simulink model "W02_Base_Map_PB_cs"  (R2019a)
settings: Solver=FixedStepDiscrete  StartTime=0.0  StopTime=inf  FixedStep=1/300  RelTol=1e-3
PreLoadFcn:
  | mbxruntime.callbacks.PreLoadFcn(bdroot);
  | check_NUTS_defined
  | model_closed = 0;
  | assignin('base',['model_closed_' bdroot],false);
PostLoadFcn:
  | mbxruntime.callbacks.PostLoadFcn(bdroot);
InitFcn:
  | mbxruntime.callbacks.InitFcn(bdroot);
StartFcn:
  | mbxruntime.callbacks.StartFcn(bdroot);
StopFcn:
  | mbxruntime.callbacks.StopFcn(bdroot);;
  | 
model workspace: external: MAT-File .\W02_Base_Map_PB_cs_hws.mat (data not in the file)
undefined symbols (not defined in the file or in its folder): DiscIntNeverNeededParam, Header, InitImageOutputDir, mbxruntime, Orientation, Pose, Poses, Poses_SL_Info, Position, tabledata
libraries: PBCSimulinkLibrary x57, simulink_extras x9, PreScanSimulinkLibrary x6, robotlib x6, PreScanUsefulBlocks x4, sharedtransform x3, aerolibutil x2, visionconversions x1, visionsinks x1
(part 4 of 7)

== system W02_Base_Map_PB_cs/TrafficLightRoadSideNL_7 ==
  note: Light SPD Resources
      |
      |  0: CIE_A_standard_incandescent_illuminant.txt
      |  1: CIE_A_standard_incandescent_illuminant.txt_x_R255_G191_B000.txt
      |  2: CIE_A_standard_incandescent_illuminant.txt_x_R583_G047_B000.txt
      |  3: CIE_F12_standard_fluorescent_illuminant.txt
      |  4: Illuminant_D65.txt
      |  5: Light_SPD_H1_12_8V_Filament.txt
      |  6: Light_SPD_H1_13_2V_Filament.txt
      |  7: Light_SPD_H11_12V_Filament.txt
      |  8: Light_SPD_H7_12_8V_Filament.txt
      |  9: Light_SPD_H7_13_2V_Filament.txt
      | 10: Light_SPD_H8_13_2V_Filament.txt
      | 11: Light_SPD_Halogen.txt
      | 12: Light_SPD_High_Power_LED.txt
      | 13: Light_SPD_HPS_High_Pressure_Sodium.txt
      | 14: Light_SPD_incandescent_traffic_signal_amber.txt
      | 15: Light_SPD_incandescent_traffic_signal_green.txt
      | 16: Light_SPD_incandescent_traffic_signal_red.txt
      | 17: Light_SPD_LED_D1S_HID.txt
      | 18: Light_SPD_LED_traffic_signal_amber.txt
      | 19: Light_SPD_LED_traffic_signal_green.txt
      | 20: Light_SPD_LED_traffic_signal_red.txt
      | 21: Light_SPD_LPS_Low_Pressure_Sodium.txt
      | 22: Light_SPD_Mercury.txt
      | 23: Light_SPD_Reddish_Neon_Sign.txt
      | 24: Noma_Twister_Blue_13W_120V.txt
      | 25: Philips_Blue_Golite_P1_Apollo_1750Lux.txt
      | 26: SPD_flat_1.0.txt
  note: Light SPD Resources
  Ground_1 : Ground
  Ground_2 : Ground
  Ground_3 : Ground
  TrafficLightRoadSideNL_7_Casing.LightGreen_Control_Mux : Subsystem  Tag=mux/plugin/LightSignals
  TrafficLightRoadSideNL_7_Casing.LightGreen_Power : Constant  Tag=TrafficLightRoadSideNL_7_Casing.LightGreen_Power  Value=0
  TrafficLightRoadSideNL_7_Casing.LightGreen_SPDIndex : Constant  Tag=TrafficLightRoadSideNL_7_Casing.LightGreen_SPDIndex  Value=15
  TrafficLightRoadSideNL_7_Casing.LightOrange_Control_Mux : Subsystem  Tag=mux/plugin/LightSignals
  TrafficLightRoadSideNL_7_Casing.LightOrange_Power : Constant  Tag=TrafficLightRoadSideNL_7_Casing.LightOrange_Power  Value=0
  TrafficLightRoadSideNL_7_Casing.LightOrange_SPDIndex : Constant  Tag=TrafficLightRoadSideNL_7_Casing.LightOrange_SPDIndex  Value=14
  TrafficLightRoadSideNL_7_Casing.LightRed_Control_Mux : Subsystem  Tag=mux/plugin/LightSignals
  TrafficLightRoadSideNL_7_Casing.LightRed_Power : Constant  Tag=TrafficLightRoadSideNL_7_Casing.LightRed_Power  Value=0
  TrafficLightRoadSideNL_7_Casing.LightRed_SPDIndex : Constant  Tag=TrafficLightRoadSideNL_7_Casing.LightRed_SPDIndex  Value=16
  VISUCasingLights_Mux : Subsystem  Tag=mux/VisuCasingLights  mask(PreScan User Interface: VisuTrafficLight){}
      mask help:
      | The VisuTrafficLight block provides a way to animate traffic lights: switch on and off individual lights.
      |
      | For more information, please click Help.
      mask Help: eval('openHelp(731)')
  VISUCasingLights_TrafficLightRoadSideNL_7 : Outport  Tag=outport/VisuCasingLights  SampleTime=1/300
  TrafficLightRoadSideNL_7_Casing.LightRed_Control : Outport  Tag=outport/plugin/sfun_PBCLight  Port=2  OutDataTypeStr=Bus: PRESCAN_PBCLIGHT_DATA  PortDimensions=1  SampleTime=0.05
  TrafficLightRoadSideNL_7_Casing.LightOrange_Control : Outport  Tag=outport/plugin/sfun_PBCLight  Port=3  OutDataTypeStr=Bus: PRESCAN_PBCLIGHT_DATA  PortDimensions=1  SampleTime=0.05
  TrafficLightRoadSideNL_7_Casing.LightGreen_Control : Outport  Tag=outport/plugin/sfun_PBCLight  Port=4  OutDataTypeStr=Bus: PRESCAN_PBCLIGHT_DATA  PortDimensions=1  SampleTime=0.05
  wires:
  VISUCasingLights_Mux/1(VISUCasingLights_TrafficLightRoadSideNL_7) -> VISUCasingLights_TrafficLightRoadSideNL_7/1
  TrafficLightRoadSideNL_7_Casing.LightRed_Control_Mux/1(Bus) -> TrafficLightRoadSideNL_7_Casing.LightRed_Control/1
  TrafficLightRoadSideNL_7_Casing.LightRed_SPDIndex/1 -> TrafficLightRoadSideNL_7_Casing.LightRed_Control_Mux/1(SPDIndex [-])
  TrafficLightRoadSideNL_7_Casing.LightRed_Power/1 -> TrafficLightRoadSideNL_7_Casing.LightRed_Control_Mux/2(Power [W])
  TrafficLightRoadSideNL_7_Casing.LightOrange_Control_Mux/1(Bus) -> TrafficLightRoadSideNL_7_Casing.LightOrange_Control/1
  TrafficLightRoadSideNL_7_Casing.LightOrange_SPDIndex/1 -> TrafficLightRoadSideNL_7_Casing.LightOrange_Control_Mux/1(SPDIndex [-])
  TrafficLightRoadSideNL_7_Casing.LightOrange_Power/1 -> TrafficLightRoadSideNL_7_Casing.LightOrange_Control_Mux/2(Power [W])
  TrafficLightRoadSideNL_7_Casing.LightGreen_Control_Mux/1(Bus) -> TrafficLightRoadSideNL_7_Casing.LightGreen_Control/1
  TrafficLightRoadSideNL_7_Casing.LightGreen_SPDIndex/1 -> TrafficLightRoadSideNL_7_Casing.LightGreen_Control_Mux/1(SPDIndex [-])
  TrafficLightRoadSideNL_7_Casing.LightGreen_Power/1 -> TrafficLightRoadSideNL_7_Casing.LightGreen_Control_Mux/2(Power [W])
  Ground_1/1 -> VISUCasingLights_Mux/1(Green [-])
  Ground_2/1 -> VISUCasingLights_Mux/2(Orange [-])
  Ground_3/1 -> VISUCasingLights_Mux/3(Red [-])

== system W02_Base_Map_PB_cs/TrafficLightRoadSideNL_7_Casing.LightGreen_Control ==
  TrafficLightRoadSideNL_7_Casing.LightGreen_Control : Inport  Tag=inport/plugin/sfun_PBCLight  OutDataTypeStr=Bus: PRESCAN_PBCLIGHT_DATA  PortDimensions=1  SampleTime=0.05  BusOutputAsStruct=on
  Actuator : S-Function  LoadFcn=addpath 'C:/Program Files/Simcenter Prescan/Prescan_2019.2/Plugins/PBCameraPlugin/matlab';addpath 'C:/Program Files/Simcenter Prescan/Prescan_2019.2/Plugins/PBCameraPlugin/bin';load('PreScanPBCLightData.mat');  FunctionName=sfun_PBCLight  Parameters=lightID, timestepMask  SFunctionDeploymentMode=off  EnableBusSupport=off  mask(Physics Based Camera plugin block){lightID=17, timestepMask=0.05}
      mask prompts: lightID "Light ID:"; timestepMask "MATLAB timestep:"
      mask help: Light Control I/O
      mask Help: eval('openHelp(6500)')
      mask Display: image(imread('ico_PBCControl.png'))
  wires:
  TrafficLightRoadSideNL_7_Casing.LightGreen_Control/1 -> Actuator/1

== system W02_Base_Map_PB_cs/TrafficLightRoadSideNL_7_Casing.LightOrange_Control ==
  TrafficLightRoadSideNL_7_Casing.LightOrange_Control : Inport  Tag=inport/plugin/sfun_PBCLight  OutDataTypeStr=Bus: PRESCAN_PBCLIGHT_DATA  PortDimensions=1  SampleTime=0.05  BusOutputAsStruct=on
  Actuator : S-Function  LoadFcn=addpath 'C:/Program Files/Simcenter Prescan/Prescan_2019.2/Plugins/PBCameraPlugin/matlab';addpath 'C:/Program Files/Simcenter Prescan/Prescan_2019.2/Plugins/PBCameraPlugin/bin';load('PreScanPBCLightData.mat');  FunctionName=sfun_PBCLight  Parameters=lightID, timestepMask  SFunctionDeploymentMode=off  EnableBusSupport=off  mask(Physics Based Camera plugin block){lightID=16, timestepMask=0.05}
      mask prompts: lightID "Light ID:"; timestepMask "MATLAB timestep:"
      mask help: Light Control I/O
      mask Help: eval('openHelp(6500)')
      mask Display: image(imread('ico_PBCControl.png'))
  wires:
  TrafficLightRoadSideNL_7_Casing.LightOrange_Control/1 -> Actuator/1

== system W02_Base_Map_PB_cs/TrafficLightRoadSideNL_7_Casing.LightRed_Control ==
  TrafficLightRoadSideNL_7_Casing.LightRed_Control : Inport  Tag=inport/plugin/sfun_PBCLight  OutDataTypeStr=Bus: PRESCAN_PBCLIGHT_DATA  PortDimensions=1  SampleTime=0.05  BusOutputAsStruct=on
  Actuator : S-Function  LoadFcn=addpath 'C:/Program Files/Simcenter Prescan/Prescan_2019.2/Plugins/PBCameraPlugin/matlab';addpath 'C:/Program Files/Simcenter Prescan/Prescan_2019.2/Plugins/PBCameraPlugin/bin';load('PreScanPBCLightData.mat');  FunctionName=sfun_PBCLight  Parameters=lightID, timestepMask  SFunctionDeploymentMode=off  EnableBusSupport=off  mask(Physics Based Camera plugin block){lightID=15, timestepMask=0.05}
      mask prompts: lightID "Light ID:"; timestepMask "MATLAB timestep:"
      mask help: Light Control I/O
      mask Help: eval('openHelp(6500)')
      mask Display: image(imread('ico_PBCControl.png'))
  wires:
  TrafficLightRoadSideNL_7_Casing.LightRed_Control/1 -> Actuator/1

== system W02_Base_Map_PB_cs/TrafficLightRoadSideNL_8 ==
  note: Light SPD Resources
      |
      |  0: CIE_A_standard_incandescent_illuminant.txt
      |  1: CIE_A_standard_incandescent_illuminant.txt_x_R255_G191_B000.txt
      |  2: CIE_A_standard_incandescent_illuminant.txt_x_R583_G047_B000.txt
      |  3: CIE_F12_standard_fluorescent_illuminant.txt
      |  4: Illuminant_D65.txt
      |  5: Light_SPD_H1_12_8V_Filament.txt
      |  6: Light_SPD_H1_13_2V_Filament.txt
      |  7: Light_SPD_H11_12V_Filament.txt
      |  8: Light_SPD_H7_12_8V_Filament.txt
      |  9: Light_SPD_H7_13_2V_Filament.txt
      | 10: Light_SPD_H8_13_2V_Filament.txt
      | 11: Light_SPD_Halogen.txt
      | 12: Light_SPD_High_Power_LED.txt
      | 13: Light_SPD_HPS_High_Pressure_Sodium.txt
      | 14: Light_SPD_incandescent_traffic_signal_amber.txt
      | 15: Light_SPD_incandescent_traffic_signal_green.txt
      | 16: Light_SPD_incandescent_traffic_signal_red.txt
      | 17: Light_SPD_LED_D1S_HID.txt
      | 18: Light_SPD_LED_traffic_signal_amber.txt
      | 19: Light_SPD_LED_traffic_signal_green.txt
      | 20: Light_SPD_LED_traffic_signal_red.txt
      | 21: Light_SPD_LPS_Low_Pressure_Sodium.txt
      | 22: Light_SPD_Mercury.txt
      | 23: Light_SPD_Reddish_Neon_Sign.txt
      | 24: Noma_Twister_Blue_13W_120V.txt
      | 25: Philips_Blue_Golite_P1_Apollo_1750Lux.txt
      | 26: SPD_flat_1.0.txt
  note: Light SPD Resources
  Ground_1 : Ground
  Ground_2 : Ground
  Ground_3 : Ground
  TrafficLightRoadSideNL_8_Casing.LightGreen_Control_Mux : Subsystem  Tag=mux/plugin/LightSignals
  TrafficLightRoadSideNL_8_Casing.LightGreen_Power : Constant  Tag=TrafficLightRoadSideNL_8_Casing.LightGreen_Power  Value=0
  TrafficLightRoadSideNL_8_Casing.LightGreen_SPDIndex : Constant  Tag=TrafficLightRoadSideNL_8_Casing.LightGreen_SPDIndex  Value=15
  TrafficLightRoadSideNL_8_Casing.LightOrange_Control_Mux : Subsystem  Tag=mux/plugin/LightSignals
  TrafficLightRoadSideNL_8_Casing.LightOrange_Power : Constant  Tag=TrafficLightRoadSideNL_8_Casing.LightOrange_Power  Value=0
  TrafficLightRoadSideNL_8_Casing.LightOrange_SPDIndex : Constant  Tag=TrafficLightRoadSideNL_8_Casing.LightOrange_SPDIndex  Value=14
  TrafficLightRoadSideNL_8_Casing.LightRed_Control_Mux : Subsystem  Tag=mux/plugin/LightSignals
  TrafficLightRoadSideNL_8_Casing.LightRed_Power : Constant  Tag=TrafficLightRoadSideNL_8_Casing.LightRed_Power  Value=0
  TrafficLightRoadSideNL_8_Casing.LightRed_SPDIndex : Constant  Tag=TrafficLightRoadSideNL_8_Casing.LightRed_SPDIndex  Value=16
  VISUCasingLights_Mux : Subsystem  Tag=mux/VisuCasingLights  mask(PreScan User Interface: VisuTrafficLight){}
      mask help:
      | The VisuTrafficLight block provides a way to animate traffic lights: switch on and off individual lights.
      |
      | For more information, please click Help.
      mask Help: eval('openHelp(731)')
  VISUCasingLights_TrafficLightRoadSideNL_8 : Outport  Tag=outport/VisuCasingLights  SampleTime=1/300
  TrafficLightRoadSideNL_8_Casing.LightRed_Control : Outport  Tag=outport/plugin/sfun_PBCLight  Port=2  OutDataTypeStr=Bus: PRESCAN_PBCLIGHT_DATA  PortDimensions=1  SampleTime=0.05
  TrafficLightRoadSideNL_8_Casing.LightOrange_Control : Outport  Tag=outport/plugin/sfun_PBCLight  Port=3  OutDataTypeStr=Bus: PRESCAN_PBCLIGHT_DATA  PortDimensions=1  SampleTime=0.05
  TrafficLightRoadSideNL_8_Casing.LightGreen_Control : Outport  Tag=outport/plugin/sfun_PBCLight  Port=4  OutDataTypeStr=Bus: PRESCAN_PBCLIGHT_DATA  PortDimensions=1  SampleTime=0.05
  wires:
  VISUCasingLights_Mux/1(VISUCasingLights_TrafficLightRoadSideNL_8) -> VISUCasingLights_TrafficLightRoadSideNL_8/1
  TrafficLightRoadSideNL_8_Casing.LightRed_Control_Mux/1(Bus) -> TrafficLightRoadSideNL_8_Casing.LightRed_Control/1
  TrafficLightRoadSideNL_8_Casing.LightRed_SPDIndex/1 -> TrafficLightRoadSideNL_8_Casing.LightRed_Control_Mux/1(SPDIndex [-])
  TrafficLightRoadSideNL_8_Casing.LightRed_Power/1 -> TrafficLightRoadSideNL_8_Casing.LightRed_Control_Mux/2(Power [W])
  TrafficLightRoadSideNL_8_Casing.LightOrange_Control_Mux/1(Bus) -> TrafficLightRoadSideNL_8_Casing.LightOrange_Control/1
  TrafficLightRoadSideNL_8_Casing.LightOrange_SPDIndex/1 -> TrafficLightRoadSideNL_8_Casing.LightOrange_Control_Mux/1(SPDIndex [-])
  TrafficLightRoadSideNL_8_Casing.LightOrange_Power/1 -> TrafficLightRoadSideNL_8_Casing.LightOrange_Control_Mux/2(Power [W])
  TrafficLightRoadSideNL_8_Casing.LightGreen_Control_Mux/1(Bus) -> TrafficLightRoadSideNL_8_Casing.LightGreen_Control/1
  TrafficLightRoadSideNL_8_Casing.LightGreen_SPDIndex/1 -> TrafficLightRoadSideNL_8_Casing.LightGreen_Control_Mux/1(SPDIndex [-])
  TrafficLightRoadSideNL_8_Casing.LightGreen_Power/1 -> TrafficLightRoadSideNL_8_Casing.LightGreen_Control_Mux/2(Power [W])
  Ground_1/1 -> VISUCasingLights_Mux/1(Green [-])
  Ground_2/1 -> VISUCasingLights_Mux/2(Orange [-])
  Ground_3/1 -> VISUCasingLights_Mux/3(Red [-])

== system W02_Base_Map_PB_cs/TrafficLightRoadSideNL_8_Casing.LightGreen_Control ==
  TrafficLightRoadSideNL_8_Casing.LightGreen_Control : Inport  Tag=inport/plugin/sfun_PBCLight  OutDataTypeStr=Bus: PRESCAN_PBCLIGHT_DATA  PortDimensions=1  SampleTime=0.05  BusOutputAsStruct=on
  Actuator : S-Function  LoadFcn=addpath 'C:/Program Files/Simcenter Prescan/Prescan_2019.2/Plugins/PBCameraPlugin/matlab';addpath 'C:/Program Files/Simcenter Prescan/Prescan_2019.2/Plugins/PBCameraPlugin/bin';load('PreScanPBCLightData.mat');  FunctionName=sfun_PBCLight  Parameters=lightID, timestepMask  SFunctionDeploymentMode=off  EnableBusSupport=off  mask(Physics Based Camera plugin block){lightID=20, timestepMask=0.05}
      mask prompts: lightID "Light ID:"; timestepMask "MATLAB timestep:"
      mask help: Light Control I/O
      mask Help: eval('openHelp(6500)')
      mask Display: image(imread('ico_PBCControl.png'))
  wires:
  TrafficLightRoadSideNL_8_Casing.LightGreen_Control/1 -> Actuator/1

== system W02_Base_Map_PB_cs/TrafficLightRoadSideNL_8_Casing.LightOrange_Control ==
  TrafficLightRoadSideNL_8_Casing.LightOrange_Control : Inport  Tag=inport/plugin/sfun_PBCLight  OutDataTypeStr=Bus: PRESCAN_PBCLIGHT_DATA  PortDimensions=1  SampleTime=0.05  BusOutputAsStruct=on
  Actuator : S-Function  LoadFcn=addpath 'C:/Program Files/Simcenter Prescan/Prescan_2019.2/Plugins/PBCameraPlugin/matlab';addpath 'C:/Program Files/Simcenter Prescan/Prescan_2019.2/Plugins/PBCameraPlugin/bin';load('PreScanPBCLightData.mat');  FunctionName=sfun_PBCLight  Parameters=lightID, timestepMask  SFunctionDeploymentMode=off  EnableBusSupport=off  mask(Physics Based Camera plugin block){lightID=19, timestepMask=0.05}
      mask prompts: lightID "Light ID:"; timestepMask "MATLAB timestep:"
      mask help: Light Control I/O
      mask Help: eval('openHelp(6500)')
      mask Display: image(imread('ico_PBCControl.png'))
  wires:
  TrafficLightRoadSideNL_8_Casing.LightOrange_Control/1 -> Actuator/1

== system W02_Base_Map_PB_cs/TrafficLightRoadSideNL_8_Casing.LightRed_Control ==
  TrafficLightRoadSideNL_8_Casing.LightRed_Control : Inport  Tag=inport/plugin/sfun_PBCLight  OutDataTypeStr=Bus: PRESCAN_PBCLIGHT_DATA  PortDimensions=1  SampleTime=0.05  BusOutputAsStruct=on
  Actuator : S-Function  LoadFcn=addpath 'C:/Program Files/Simcenter Prescan/Prescan_2019.2/Plugins/PBCameraPlugin/matlab';addpath 'C:/Program Files/Simcenter Prescan/Prescan_2019.2/Plugins/PBCameraPlugin/bin';load('PreScanPBCLightData.mat');  FunctionName=sfun_PBCLight  Parameters=lightID, timestepMask  SFunctionDeploymentMode=off  EnableBusSupport=off  mask(Physics Based Camera plugin block){lightID=18, timestepMask=0.05}
      mask prompts: lightID "Light ID:"; timestepMask "MATLAB timestep:"
      mask help: Light Control I/O
      mask Help: eval('openHelp(6500)')
      mask Display: image(imread('ico_PBCControl.png'))
  wires:
  TrafficLightRoadSideNL_8_Casing.LightRed_Control/1 -> Actuator/1

== system W02_Base_Map_PB_cs/VISUCasingLights_TrafficLightRoadSideNL_1 ==
  VISUCasingLights_TrafficLightRoadSideNL_1 : Inport  Tag=inport/VisuCasingLights  SampleTime=1/300  BusOutputAsStruct=on
  Actuator : Subsystem  mask(PreScan Sink Block: VisuTrafficLight){UniqueID=646, ColorsObjectQuery=, Colors=[]}
      mask prompts: UniqueID "Parent Unique Identifier"; ColorsObjectQuery "Query for Color Object"; Colors "Matrix of colors"
      mask help:
      | The VisuTrafficLight block provides a way to animate traffic lights: switch on and off individual lights.
      |
      | For more information, please click Help.
      mask Help: eval('openHelp(731)')
      mask Display: image(imread('TrafficLightCasing.png'))
  wires:
  VISUCasingLights_TrafficLightRoadSideNL_1/1 -> Actuator/1(VISUCasingLights_TrafficLightRoadSideNL_1)

== system W02_Base_Map_PB_cs/VISUCasingLights_TrafficLightRoadSideNL_2 ==
  VISUCasingLights_TrafficLightRoadSideNL_2 : Inport  Tag=inport/VisuCasingLights  SampleTime=1/300  BusOutputAsStruct=on
  Actuator : Subsystem  mask(PreScan Sink Block: VisuTrafficLight){UniqueID=647, ColorsObjectQuery=, Colors=[]}
      mask prompts: UniqueID "Parent Unique Identifier"; ColorsObjectQuery "Query for Color Object"; Colors "Matrix of colors"
      mask help:
      | The VisuTrafficLight block provides a way to animate traffic lights: switch on and off individual lights.
      |
      | For more information, please click Help.
      mask Help: eval('openHelp(731)')
      mask Display: image(imread('TrafficLightCasing.png'))
  wires:
  VISUCasingLights_TrafficLightRoadSideNL_2/1 -> Actuator/1(VISUCasingLights_TrafficLightRoadSideNL_2)

== system W02_Base_Map_PB_cs/VISUCasingLights_TrafficLightRoadSideNL_3 ==
  VISUCasingLights_TrafficLightRoadSideNL_3 : Inport  Tag=inport/VisuCasingLights  SampleTime=1/300  BusOutputAsStruct=on
  Actuator : Subsystem  mask(PreScan Sink Block: VisuTrafficLight){UniqueID=649, ColorsObjectQuery=, Colors=[]}
      mask prompts: UniqueID "Parent Unique Identifier"; ColorsObjectQuery "Query for Color Object"; Colors "Matrix of colors"
      mask help:
      | The VisuTrafficLight block provides a way to animate traffic lights: switch on and off individual lights.
      |
      | For more information, please click Help.
      mask Help: eval('openHelp(731)')
      mask Display: image(imread('TrafficLightCasing.png'))
  wires:
  VISUCasingLights_TrafficLightRoadSideNL_3/1 -> Actuator/1(VISUCasingLights_TrafficLightRoadSideNL_3)

== system W02_Base_Map_PB_cs/VISUCasingLights_TrafficLightRoadSideNL_4 ==
  VISUCasingLights_TrafficLightRoadSideNL_4 : Inport  Tag=inport/VisuCasingLights  SampleTime=1/300  BusOutputAsStruct=on
  Actuator : Subsystem  mask(PreScan Sink Block: VisuTrafficLight){UniqueID=650, ColorsObjectQuery=, Colors=[]}
      mask prompts: UniqueID "Parent Unique Identifier"; ColorsObjectQuery "Query for Color Object"; Colors "Matrix of colors"
      mask help:
      | The VisuTrafficLight block provides a way to animate traffic lights: switch on and off individual lights.
      |
      | For more information, please click Help.
      mask Help: eval('openHelp(731)')
      mask Display: image(imread('TrafficLightCasing.png'))
  wires:
  VISUCasingLights_TrafficLightRoadSideNL_4/1 -> Actuator/1(VISUCasingLights_TrafficLightRoadSideNL_4)

== system W02_Base_Map_PB_cs/VISUCasingLights_TrafficLightRoadSideNL_5 ==
  VISUCasingLights_TrafficLightRoadSideNL_5 : Inport  Tag=inport/VisuCasingLights  SampleTime=1/300  BusOutputAsStruct=on
  Actuator : Subsystem  mask(PreScan Sink Block: VisuTrafficLight){UniqueID=651, ColorsObjectQuery=, Colors=[]}
      mask prompts: UniqueID "Parent Unique Identifier"; ColorsObjectQuery "Query for Color Object"; Colors "Matrix of colors"
      mask help:
      | The VisuTrafficLight block provides a way to animate traffic lights: switch on and off individual lights.
      |
      | For more information, please click Help.
      mask Help: eval('openHelp(731)')
      mask Display: image(imread('TrafficLightCasing.png'))
  wires:
  VISUCasingLights_TrafficLightRoadSideNL_5/1 -> Actuator/1(VISUCasingLights_TrafficLightRoadSideNL_5)

== system W02_Base_Map_PB_cs/VISUCasingLights_TrafficLightRoadSideNL_6 ==
  VISUCasingLights_TrafficLightRoadSideNL_6 : Inport  Tag=inport/VisuCasingLights  SampleTime=1/300  BusOutputAsStruct=on
  Actuator : Subsystem  mask(PreScan Sink Block: VisuTrafficLight){UniqueID=10446, ColorsObjectQuery=, Colors=[]}
      mask prompts: UniqueID "Parent Unique Identifier"; ColorsObjectQuery "Query for Color Object"; Colors "Matrix of colors"
      mask help:
      | The VisuTrafficLight block provides a way to animate traffic lights: switch on and off individual lights.
      |
      | For more information, please click Help.
      mask Help: eval('openHelp(731)')
      mask Display: image(imread('TrafficLightCasing.png'))
  wires:
  VISUCasingLights_TrafficLightRoadSideNL_6/1 -> Actuator/1(VISUCasingLights_TrafficLightRoadSideNL_6)

== system W02_Base_Map_PB_cs/VISUCasingLights_TrafficLightRoadSideNL_7 ==
  VISUCasingLights_TrafficLightRoadSideNL_7 : Inport  Tag=inport/VisuCasingLights  SampleTime=1/300  BusOutputAsStruct=on
  Actuator : Subsystem  mask(PreScan Sink Block: VisuTrafficLight){UniqueID=653, ColorsObjectQuery=, Colors=[]}
      mask prompts: UniqueID "Parent Unique Identifier"; ColorsObjectQuery "Query for Color Object"; Colors "Matrix of colors"
      mask help:
      | The VisuTrafficLight block provides a way to animate traffic lights: switch on and off individual lights.
      |
      | For more information, please click Help.
      mask Help: eval('openHelp(731)')
      mask Display: image(imread('TrafficLightCasing.png'))
  wires:
  VISUCasingLights_TrafficLightRoadSideNL_7/1 -> Actuator/1(VISUCasingLights_TrafficLightRoadSideNL_7)

== system W02_Base_Map_PB_cs/VISUCasingLights_TrafficLightRoadSideNL_8 ==
  VISUCasingLights_TrafficLightRoadSideNL_8 : Inport  Tag=inport/VisuCasingLights  SampleTime=1/300  BusOutputAsStruct=on
  Actuator : Subsystem  mask(PreScan Sink Block: VisuTrafficLight){UniqueID=654, ColorsObjectQuery=, Colors=[]}
      mask prompts: UniqueID "Parent Unique Identifier"; ColorsObjectQuery "Query for Color Object"; Colors "Matrix of colors"
      mask help:
      | The VisuTrafficLight block provides a way to animate traffic lights: switch on and off individual lights.
      |
      | For more information, please click Help.
      mask Help: eval('openHelp(731)')
      mask Display: image(imread('TrafficLightCasing.png'))
  wires:
  VISUCasingLights_TrafficLightRoadSideNL_8/1 -> Actuator/1(VISUCasingLights_TrafficLightRoadSideNL_8)

== system W02_Base_Map_PB_cs/pose_otheCar ==
  In1 : Inport
  Enable : EnablePort
  Add5 : Sum
  Assignment : Assignment  OutputInitialize=Specify size for each dimension in table  DiagnosticForDimensions=Warning  IndexOptions=Starting index (dialog)  Indices=1  OutputSizes=1
  Assignment2 : Assignment  OutputInitialize=Specify size for each dimension in table  DiagnosticForDimensions=Warning  IndexOptions=Starting index (dialog)  Indices=1  OutputSizes=1000
  Blank Message1 : robotlib/Blank Message  messageClass=Message  entityType=geometry_msgs/PoseArray  messageType=geometry_msgs/PoseArray  SampleTime=inf
      settings: SourceProductBaseCode=RO
  Bus Assignment3 : BusAssignment  AssignedSignals=Header.Seq,Header.FrameId,Header.FrameId_SL_Info.CurrentLength,Poses,Poses_SL_Info.CurrentLength
  Bus Selector : BusSelector  OutputSignals=Poses
  Bus Selector2 : BusSelector  OutputSignals=Header.FrameId
  Constant24 : Constant  OutDataTypeStr=uint32
  Constant25 : Constant  Value=uint8(['map'])
  Memory2 : Memory  InheritSampleTime=on
  Publish2 : robotlib/Publish  topicSource=Specify your own  topic=/pose_otherCar  messageType=geometry_msgs/PoseArray  messageQueueLength=1
      settings: SourceProductBaseCode=RO
  Width : Width  DataType=uint32
  Width5 : Width  DataType=uint32
  wires:
  Constant24/1 -> Add5/2
  Memory2/1 -> Add5/1
  Add5/1 -> Bus Assignment3/2, Memory2/1
  Width5/1 -> Bus Assignment3/4
  Assignment/1 -> Bus Assignment3/5, Width/1
  Width/1 -> Bus Assignment3/6
  Bus Selector/1 -> Assignment/1  "<Poses>"
  In1/1 -> Assignment/2
  Bus Assignment3/1 -> Publish2/1
  Constant25/1 -> Assignment2/2
  Assignment2/1 -> Bus Assignment3/3, Width5/1
  Bus Selector2/1 -> Assignment2/1  "<FrameId>"
  Blank Message1/1 -> Bus Selector/1, Bus Selector2/1, Bus Assignment3/1

== system W02_Base_Map_PB_cs/tl_camera ==
  Sensor : S-Function  FunctionName=sfun_Camera  Parameters=sensorID, dataWidth, dataHeight, channelsPerImage, numberOfImages, timestep  SFunctionDeploymentMode=off  EnableBusSupport=off  mask(PreScan Source Block: Camera Sensor){sensorID=12017, dataWidth=720, dataHeight=2880, channelsPerImage=3, numberOfImages=1, timestep=1/20}
      mask prompts: sensorID "Sensor ID"; dataWidth "Data width"; dataHeight "Data Height"; channelsPerImage "Channels per image"; numberOfImages "Number of images"; timestep "MATLAB timestep:"
      mask help: The Camera Sensor provides a color or monochrome image.
      mask Help: eval('openHelp(457)')
      mask Display: image(imread('CameraSensor.png'))
  tl_camera : Outport  Tag=outport/Camera/CameraSensor  OutDataTypeStr=uint8  SampleTime=1/20
  wires:
  Sensor/1 -> tl_camera/1

== system W02_Base_Map_PB_cs/BMW_X5_SUV_1/Car_Pose ==
  In1 : Inport
  In2 : Inport  Port=2
  In3 : Inport  Port=3
  In4 : Inport  Port=4
  In5 : Inport  Port=5
  In6 : Inport  Port=6
  Data Type Conversion : DataTypeConversion
  Data Type Conversion1 : DataTypeConversion
  Data Type Conversion2 : DataTypeConversion
  Degrees to Radians1 : simulink_extras/Transformations/Degrees to Radians
  Degrees to Radians2 : simulink_extras/Transformations/Degrees to Radians
  Degrees to Radians5 : simulink_extras/Transformations/Degrees to Radians
  Mux : Mux
  Rotation Angles to Quaternions : sharedtransform/Rotation Angles to Quaternions  rotationOrder=XYZ  aMode=aMode
      settings: SourceProductName=Aerospace Blockset  SourceProductBaseCode=AE
  Vector Concatenate2 : Concatenate  NumInputs=3
  Out1 : Outport
  wires:
  Mux/1 -> Out1/1
  Rotation Angles to Quaternions/1 -> Mux/4
  Data Type Conversion2/1 -> Mux/3
  Data Type Conversion1/1 -> Mux/2
  Data Type Conversion/1 -> Mux/1
  In6/1 -> Degrees to Radians2/1
  In5/1 -> Degrees to Radians1/1
  In4/1 -> Degrees to Radians5/1
  In3/1 -> Data Type Conversion2/1
  In2/1 -> Data Type Conversion1/1
  In1/1 -> Data Type Conversion/1
  Degrees to Radians2/1 -> Vector Concatenate2/3
  Vector Concatenate2/1 -> Rotation Angles to Quaternions/1
  Degrees to Radians5/1 -> Vector Concatenate2/1
  Degrees to Radians1/1 -> Vector Concatenate2/2

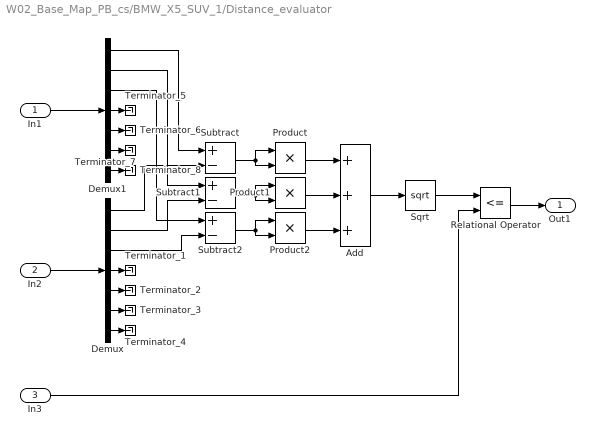
== system W02_Base_Map_PB_cs/BMW_X5_SUV_1/Distance_evaluator ==
  In1 : Inport
  In2 : Inport  Port=2
  In3 : Inport  Port=3
  Add : Sum  Inputs=3
  Demux : Demux  Outputs=7
  Demux1 : Demux  Outputs=7
  Product : Product
  Product1 : Product
  Product2 : Product
  Relational Operator : RelationalOperator  Operator=<=  OutDataTypeStr=boolean  RndMeth=Simplest
  Sqrt : Sqrt  SaturateOnIntegerOverflow=on
  Subtract : Sum  Inputs=+-
  Subtract1 : Sum  Inputs=+-
  Subtract2 : Sum  Inputs=+-
  Terminator_{1..8} (8 alike) : Terminator
  Out1 : Outport
  wires:
  Demux1/7 -> Terminator_8/1
  Demux1/6 -> Terminator_7/1
  Demux1/5 -> Terminator_6/1
  Demux1/4 -> Terminator_5/1
  Demux/7 -> Terminator_4/1
  Demux/6 -> Terminator_3/1
  Demux/5 -> Terminator_2/1
  Demux/4 -> Terminator_1/1
  In3/1 -> Relational Operator/2
  Sqrt/1 -> Relational Operator/1
  Add/1 -> Sqrt/1
  Product2/1 -> Add/3
  Product1/1 -> Add/2
  Product/1 -> Add/1
  Subtract2/1 -> Product2/2, Product2/1
  Subtract1/1 -> Product1/2, Product1/1
  Subtract/1 -> Product/2, Product/1
  Demux/3 -> Subtract2/2
  Demux/2 -> Subtract1/2
  Demux/1 -> Subtract/2
  Demux1/3 -> Subtract2/1
  Demux1/2 -> Subtract1/1
  Demux1/1 -> Subtract/1
  In2/1 -> Demux/1
  In1/1 -> Demux1/1
  Relational Operator/1 -> Out1/1

== system W02_Base_Map_PB_cs/BMW_X5_SUV_1/Dynamics_Empty ==
  note: For state mode 'Dynamic' positions
      | are not taken into account, as they
      | are computed by integrating velocity.
      | Click annotation for Help.
  Ground_{1..9} (9 alike) : Ground
  MuxState : Subsystem  Tag=mux/State  mask(Empty Dynamics State Block){positioningmode=on, TimeStep=1/300}
      mask prompts: positioningmode "Positioning Mode"; TimeStep "Auto Assigned: Time Step [s]"
      mask help:
      | Build the state of an actor based on user input.
      | The user can either use positioning mode or dynamics mode.
      | - When using positioning mode the position and orientation of the actor are set directly based on the input. Expected input is relative to the initial position and orientation of the actor. It's also possible to specify the velocity of the actor, though this input isn't used, only passed on.
      | - When using dynamics mode the position input is ignored. Expected input is velocity and orientation. The velocity is relative the current orientation of the actor, while orientation is relative to its initial orientation. The position of the actor is calculated based on the velocity and orientation given.
      settings: DeleteFcn=PreScanBlockDeleteFcn;
  STATE_BMW_X5_SUV_1 : Subsystem  Tag=mux/StatePort  Priority=0  LoadFcn=load PrescanStateActuatorData  mask(PreScan Sink Block: State){x0=34.1533, y0=171.1318, z0=0.69, Roll0=0, Pitch0=0, Yaw0=359.6719, TimeStep=1/300}
      mask prompts: x0 "Ini x-position VEHICLE wrt GLOBAL axis system [m]"; y0 "Ini y-position VEHICLE wrt GLOBAL axis system [m]"; z0 "Ini z-position VEHICLE wrt GLOBAL axis system [m]"; Roll0 "Ini roll-angle BODY wrt VEHICLE axis system [deg]"; Pitch0 "Ini pitch-angle BODY wrt VEHICLE axis system [deg]"; Yaw0 "Ini yaw-angle VEHICLE wrt GLOBAL axis system [deg]"; TimeStep "Auto-Assigned: Upload Period [s]"
      mask help:
      | The Actor State contains a vector signal of size (9x1), containing the following signals:
      |
      | -  Position                  (x,y,z)                                     [m]
      | -  Velocity                  (vx,vy,vz)                               [m/s]
      | -  Angles                    (Roll, Pitch, Yaw)                   [rad]
      |
      | The Actor state is defined in the global axis system.
      | The state is superponed on the Initial position defined in the GUI.
      |
      | For more information, please click Help.
      settings: DeleteFcn=PreScanBlockDeleteFcn;
      mask Help: eval('openHelp(222)')
      mask Display: image(imread('State.png'))
  Sine Wave Function : Sin  Amplitude=0.1  SampleTime=0
  Terminator_1 : Terminator
  State : Outport  Tag=outport/StateOutport  SampleTime=1/300
  wires:
  MuxState/1(state) -> STATE_BMW_X5_SUV_1/1(State)
  STATE_BMW_X5_SUV_1/1(StateBus) -> State/1
  Ground_1/1 -> MuxState/1(x [m])
  Ground_2/1 -> MuxState/2(y [m])
  Ground_3/1 -> MuxState/3(z [m])
  Ground_4/1 -> MuxState/4(dx [m/s])
  Ground_5/1 -> MuxState/5(dy [m/s])
  Ground_6/1 -> MuxState/6(dz [m/s])
  Ground_7/1 -> MuxState/7(R [rad])
  Ground_8/1 -> MuxState/8(P [rad])
  Ground_9/1 -> MuxState/9(Y [rad])
  Sine Wave Function/1 -> Terminator_1/1

== system W02_Base_Map_PB_cs/BMW_X5_SUV_1/Frequency evaluator ==
  In1 : Inport
  Add : Sum  Inputs=+-
  Clock2 : Clock
  Constant : Constant
  Divide : Product  Inputs=*/
  Memory : Memory
  Relational Operator : RelationalOperator  OutDataTypeStr=boolean  RndMeth=Simplest
  Switch : Switch  Criteria=u2 > Threshold
  Out1 : Outport
  wires:
  Divide/1 -> Relational Operator/2
  Constant/1 -> Divide/1
  In1/1 -> Divide/2
  Clock2/1 -> Switch/1, Add/1
  Relational Operator/1 -> Out1/1, Switch/2
  Add/1 -> Relational Operator/1
  Switch/1 -> Memory/1
  Memory/1 -> Add/2, Switch/3

== system W02_Base_Map_PB_cs/BMW_X5_SUV_1/Frequency evaluator1 ==
  In1 : Inport
  Add : Sum  Inputs=+-
  Clock2 : Clock
  Constant : Constant
  Divide : Product  Inputs=*/
  Memory : Memory
  Relational Operator : RelationalOperator  OutDataTypeStr=boolean  RndMeth=Simplest
  Switch : Switch  Criteria=u2 > Threshold
  Out1 : Outport
  wires:
  Divide/1 -> Relational Operator/2
  Constant/1 -> Divide/1
  In1/1 -> Divide/2
  Clock2/1 -> Switch/1, Add/1
  Relational Operator/1 -> Out1/1, Switch/2
  Add/1 -> Relational Operator/1
  Switch/1 -> Memory/1
  Memory/1 -> Add/2, Switch/3

== system W02_Base_Map_PB_cs/BMW_X5_SUV_1/Frequency evaluator2 ==
  In1 : Inport
  Add : Sum  Inputs=+-
  Clock2 : Clock
  Constant : Constant
  Divide : Product  Inputs=*/
  Memory : Memory
  Relational Operator : RelationalOperator  OutDataTypeStr=boolean  RndMeth=Simplest
  Switch : Switch  Criteria=u2 > Threshold
  Out1 : Outport
  wires:
  Divide/1 -> Relational Operator/2
  Constant/1 -> Divide/1
  In1/1 -> Divide/2
  Clock2/1 -> Switch/1, Add/1
  Relational Operator/1 -> Out1/1, Switch/2
  Add/1 -> Relational Operator/1
  Switch/1 -> Memory/1
  Memory/1 -> Add/2, Switch/3

== system W02_Base_Map_PB_cs/BMW_X5_SUV_1/Frequency evaluator3 ==
  In1 : Inport
  Add : Sum  Inputs=+-
  Clock2 : Clock
  Constant : Constant
  Divide : Product  Inputs=*/
  Memory : Memory
  Relational Operator : RelationalOperator  OutDataTypeStr=boolean  RndMeth=Simplest
  Switch : Switch  Criteria=u2 > Threshold
  Out1 : Outport
  wires:
  Divide/1 -> Relational Operator/2
  Constant/1 -> Divide/1
  In1/1 -> Divide/2
  Clock2/1 -> Switch/1, Add/1
  Relational Operator/1 -> Out1/1, Switch/2
  Add/1 -> Relational Operator/1
  Switch/1 -> Memory/1
  Memory/1 -> Add/2, Switch/3

== system W02_Base_Map_PB_cs/BMW_X5_SUV_1/Frequency evaluator4 ==
  In1 : Inport
  Add : Sum  Inputs=+-
  Clock2 : Clock
  Constant : Constant
  Divide : Product  Inputs=*/
  Memory : Memory
  Relational Operator : RelationalOperator  OutDataTypeStr=boolean  RndMeth=Simplest
  Switch : Switch  Criteria=u2 > Threshold
  Out1 : Outport
  wires:
  Divide/1 -> Relational Operator/2
  Constant/1 -> Divide/1
  In1/1 -> Divide/2
  Clock2/1 -> Switch/1, Add/1
  Relational Operator/1 -> Out1/1, Switch/2
  Add/1 -> Relational Operator/1
  Switch/1 -> Memory/1
  Memory/1 -> Add/2, Switch/3

== system W02_Base_Map_PB_cs/BMW_X5_SUV_1/Frequency evaluator5 ==
  In1 : Inport
  Add : Sum  Inputs=+-
  Clock2 : Clock
  Constant : Constant
  Divide : Product  Inputs=*/
  Memory : Memory
  Relational Operator : RelationalOperator  OutDataTypeStr=boolean  RndMeth=Simplest
  Switch : Switch  Criteria=u2 > Threshold
  Out1 : Outport
  wires:
  Divide/1 -> Relational Operator/2
  Constant/1 -> Divide/1
  In1/1 -> Divide/2
  Clock2/1 -> Switch/1, Add/1
  Relational Operator/1 -> Out1/1, Switch/2
  Add/1 -> Relational Operator/1
  Switch/1 -> Memory/1
  Memory/1 -> Add/2, Switch/3

== system W02_Base_Map_PB_cs/BMW_X5_SUV_1/Frequency evaluator7 ==
  In1 : Inport
  Add : Sum  Inputs=+-
  Clock2 : Clock
  Constant : Constant
  Divide : Product  Inputs=*/
  Memory : Memory
  Relational Operator : RelationalOperator  OutDataTypeStr=boolean  RndMeth=Simplest
  Switch : Switch  Criteria=u2 > Threshold
  Out1 : Outport
  wires:
  Memory/1 -> Switch/3, Add/2
  Switch/1 -> Memory/1
  Add/1 -> Relational Operator/1
  Relational Operator/1 -> Switch/2, Out1/1
  Clock2/1 -> Add/1, Switch/1
  In1/1 -> Divide/2
  Constant/1 -> Divide/1
  Divide/1 -> Relational Operator/2

== system W02_Base_Map_PB_cs/BMW_X5_SUV_1/Lidar_1_Demux ==
  Lidar : Inport
  Bus Selector : BusSelector  OutputSignals=ActiveBeamID[-],Range[m],DopplerVelocity[ms-1],DopplerVelocityX[ms-1],DopplerVelocityY[ms-1],DopplerVelocityZ[ms-1],Theta[deg],Phi[deg],TargetID[-],TargetTypeID[-],EnergyLoss[dB],Alpha[deg],Beta[deg]  OutputAsBus=on
  ScannerSensorLegacyBusConversion : PreScanUsefulBlocks/ScannerSensorLegacyBusConversion  MAXMESSAGES=MAXMESSAGES
  Lidar Data : Outport
  wires:
  Bus Selector/1 -> Lidar Data/1
  ScannerSensorLegacyBusConversion/1 -> Bus Selector/1
  Lidar/1 -> ScannerSensorLegacyBusConversion/1

== system W02_Base_Map_PB_cs/BMW_X5_SUV_1/Lidar_2_Demux ==
  Lidar : Inport
  Bus Selector : BusSelector  OutputSignals=ActiveBeamID[-],Range[m],DopplerVelocity[ms-1],DopplerVelocityX[ms-1],DopplerVelocityY[ms-1],DopplerVelocityZ[ms-1],Theta[deg],Phi[deg],TargetID[-],TargetTypeID[-],EnergyLoss[dB],Alpha[deg],Beta[deg]  OutputAsBus=on
  ScannerSensorLegacyBusConversion : PreScanUsefulBlocks/ScannerSensorLegacyBusConversion  MAXMESSAGES=MAXMESSAGES
  Lidar Data : Outport
  wires:
  Bus Selector/1 -> Lidar Data/1
  ScannerSensorLegacyBusConversion/1 -> Bus Selector/1
  Lidar/1 -> ScannerSensorLegacyBusConversion/1

== system W02_Base_Map_PB_cs/BMW_X5_SUV_1/Lidar_3_Demux ==
  Lidar : Inport
  Bus Selector : BusSelector  OutputSignals=ActiveBeamID[-],Range[m],DopplerVelocity[ms-1],DopplerVelocityX[ms-1],DopplerVelocityY[ms-1],DopplerVelocityZ[ms-1],Theta[deg],Phi[deg],TargetID[-],TargetTypeID[-],EnergyLoss[dB],Alpha[deg],Beta[deg]  OutputAsBus=on
  ScannerSensorLegacyBusConversion : PreScanUsefulBlocks/ScannerSensorLegacyBusConversion  MAXMESSAGES=MAXMESSAGES
  Lidar Data : Outport
  wires:
  Bus Selector/1 -> Lidar Data/1
  ScannerSensorLegacyBusConversion/1 -> Bus Selector/1
  Lidar/1 -> ScannerSensorLegacyBusConversion/1

== system W02_Base_Map_PB_cs/BMW_X5_SUV_1/Lidar_4_Demux ==
  Lidar : Inport
  Bus Selector : BusSelector  OutputSignals=ActiveBeamID[-],Range[m],DopplerVelocity[ms-1],DopplerVelocityX[ms-1],DopplerVelocityY[ms-1],DopplerVelocityZ[ms-1],Theta[deg],Phi[deg],TargetID[-],TargetTypeID[-],EnergyLoss[dB],Alpha[deg],Beta[deg]  OutputAsBus=on
  ScannerSensorLegacyBusConversion : PreScanUsefulBlocks/ScannerSensorLegacyBusConversion  MAXMESSAGES=MAXMESSAGES
  Lidar Data : Outport
  wires:
  Bus Selector/1 -> Lidar Data/1
  ScannerSensorLegacyBusConversion/1 -> Bus Selector/1
  Lidar/1 -> ScannerSensorLegacyBusConversion/1

== system W02_Base_Map_PB_cs/BMW_X5_SUV_1/PhysicsBasedCameraSensor_1_PBCPose_Control_Mux ==
  Position [m] : Inport
  Orientation [rad] : Inport  Port=2
  Bus Creator1 : BusCreator  Inputs=12  OutDataTypeStr=Bus: PRESCAN_PBCPOSE_DATA  NonVirtualBus=on
  Demux{,1..3} (4 alike) : Demux  Outputs=3
  SignalChanged : PBCSimulinkLibrary/SignalChanged  SystemSampleTime=-1
  SignalChanged1 : PBCSimulinkLibrary/SignalChanged  SystemSampleTime=-1
  Bus : Outport
  wires:
  Demux1/3 -> Bus Creator1/12  "OrientationYaw"
  Demux1/2 -> Bus Creator1/11  "OrientationPitch"
  Demux1/1 -> Bus Creator1/10  "OrientationRoll"
  Demux3/3 -> Bus Creator1/9  "OrientationYawDefined"
  Demux3/2 -> Bus Creator1/8  "OrientationPitchDefined"
  Demux3/1 -> Bus Creator1/7  "OrientationRollDefined"
  Demux/3 -> Bus Creator1/6  "PositionZ"
  Demux/2 -> Bus Creator1/5  "PositionY"
  Demux/1 -> Bus Creator1/4  "PositionX"
  Demux2/3 -> Bus Creator1/3  "PositionZDefined"
  Demux2/2 -> Bus Creator1/2  "PositionYDefined"
  Demux2/1 -> Bus Creator1/1  "PositionXDefined"
  SignalChanged1/1 -> Demux3/1
  SignalChanged/1 -> Demux2/1
  Bus Creator1/1 -> Bus/1
  Position [m]/1 -> SignalChanged/1, Demux/1
  Orientation [rad]/1 -> SignalChanged1/1, Demux1/1

== system W02_Base_Map_PB_cs/BMW_X5_SUV_1/PhysicsBasedCameraSensor_1_PBC_Control_Mux ==
  IntegrationTime [s] : Inport
  DigitalGain0 [-] : Inport  Port=2
  DigitalGain1 [-] : Inport  Port=3
  DigitalGain2 [-] : Inport  Port=4
  DigitalGain3 [-] : Inport  Port=5
  AnalogGain [-] : Inport  Port=6
  InterRowIntegrationDelay [s] : Inport  Port=7
  Bus Creator1 : BusCreator  Inputs=14  OutDataTypeStr=Bus: PRESCAN_PBCCONTROL_DATA  NonVirtualBus=on
  NonNegativeSignalChanged{1..7} (7 alike) : PBCSimulinkLibrary/NonNegativeSignalChanged  SystemSampleTime=-1
  Bus : Outport
  wires:
  NonNegativeSignalChanged7/1 -> Bus Creator1/13  "InterRowIntegrationDelayDefined"
  InterRowIntegrationDelay [s]/1 -> Bus Creator1/14, NonNegativeSignalChanged7/1  "InterRowIntegrationDelay"
  NonNegativeSignalChanged6/1 -> Bus Creator1/11  "AnalogGainDefined"
  AnalogGain [-]/1 -> Bus Creator1/12, NonNegativeSignalChanged6/1  "AnalogGain"
  NonNegativeSignalChanged5/1 -> Bus Creator1/9  "DigitalGain3Defined"
  NonNegativeSignalChanged4/1 -> Bus Creator1/7  "DigitalGain2Defined"
  NonNegativeSignalChanged3/1 -> Bus Creator1/5  "DigitalGain1Defined"
  NonNegativeSignalChanged2/1 -> Bus Creator1/3  "DigitalGain0Defined"
  NonNegativeSignalChanged1/1 -> Bus Creator1/1  "IntegrationTimeDefined"
  DigitalGain3 [-]/1 -> Bus Creator1/10, NonNegativeSignalChanged5/1  "DigitalGain3"
  DigitalGain2 [-]/1 -> Bus Creator1/8, NonNegativeSignalChanged4/1  "DigitalGain2"
  DigitalGain1 [-]/1 -> Bus Creator1/6, NonNegativeSignalChanged3/1  "DigitalGain1"
  DigitalGain0 [-]/1 -> Bus Creator1/4, NonNegativeSignalChanged2/1  "DigitalGain0"
  IntegrationTime [s]/1 -> Bus Creator1/2, NonNegativeSignalChanged1/1  "IntegrationTime"
  Bus Creator1/1 -> Bus/1

== system W02_Base_Map_PB_cs/BMW_X5_SUV_1/PhysicsBasedCameraSensor_1_capture_opticsandsensor_Demux ==
  note: This block exists for legacy compatibility only
  In1 : Inport
  I : Outport
  wires:
  In1/1 -> I/1

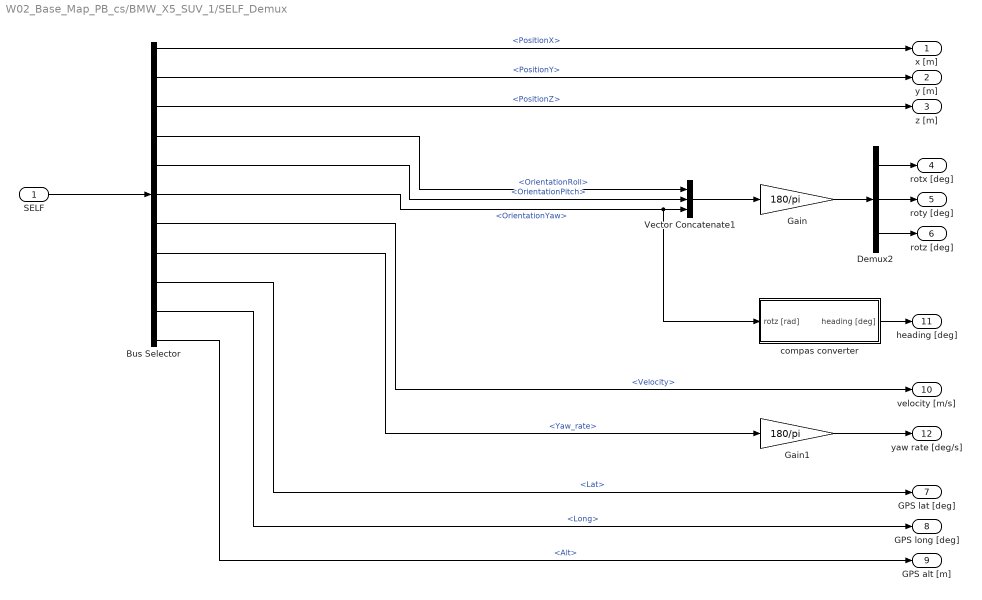
== system W02_Base_Map_PB_cs/BMW_X5_SUV_1/SELF_Demux ==
  SELF : Inport  OutDataTypeStr=Bus: PRESCAN_SELFSENSORDATA
  Bus Selector : BusSelector  OutputSignals=PositionX,PositionY,PositionZ,OrientationRoll,OrientationPitch,OrientationYaw,Velocity,Yaw_rate,Lat,Long,Alt
  Demux2 : Demux  Outputs=3
  Gain : Gain  Gain=180/pi
  Gain1 : Gain  Gain=180/pi
  Vector Concatenate1 : Concatenate  NumInputs=3
  compas converter : Subsystem
  x [m] : Outport
  y [m] : Outport  Port=2
  z [m] : Outport  Port=3
  rotx [deg] : Outport  Port=4
  roty [deg] : Outport  Port=5
  rotz [deg] : Outport  Port=6
  GPS lat [deg] : Outport  Port=7
  GPS long [deg] : Outport  Port=8
  GPS alt [m] : Outport  Port=9
  velocity [m/s] : Outport  Port=10
  heading [deg] : Outport  Port=11
  yaw rate [deg/s] : Outport  Port=12
  wires:
  Bus Selector/11 -> GPS alt [m]/1  "<Alt>"
  Bus Selector/10 -> GPS long [deg]/1  "<Long>"
  Bus Selector/9 -> GPS lat [deg]/1  "<Lat>"
  Bus Selector/8 -> Gain1/1  "<Yaw_rate>"
  Bus Selector/7 -> velocity [m/s]/1  "<Velocity>"
  Bus Selector/6 -> compas converter/1(rotz [rad]), Vector Concatenate1/3  "<OrientationYaw>"
  Bus Selector/5 -> Vector Concatenate1/2  "<OrientationPitch>"
  Bus Selector/4 -> Vector Concatenate1/1  "<OrientationRoll>"
  Vector Concatenate1/1 -> Gain/1
  Bus Selector/3 -> z [m]/1  "<PositionZ>"
  Bus Selector/2 -> y [m]/1  "<PositionY>"
  Bus Selector/1 -> x [m]/1  "<PositionX>"
  SELF/1 -> Bus Selector/1
  Gain/1 -> Demux2/1
  Demux2/1 -> rotx [deg]/1
  Demux2/2 -> roty [deg]/1
  Demux2/3 -> rotz [deg]/1
  compas converter/1(heading [deg]) -> heading [deg]/1
  Gain1/1 -> yaw rate [deg/s]/1

== system W02_Base_Map_PB_cs/BMW_X5_SUV_1/Sensor_Pose ==
  In1 : Inport
  In2 : Inport  Port=2
  In3 : Inport  Port=3
  In4 : Inport  Port=4
  Add1 : Sum
  Add2 : Sum
  Add3 : Sum
  Data Type Conversion4 : DataTypeConversion
  Demux : Demux  Outputs=7
  Demux1 : Demux  Outputs=3
  Mux : Mux
  Mux1 : Mux
  Quaternion Conjugate1 : aerolibutil/Quaternion Conjugate
      settings: SourceProductName=Aerospace Blockset  SourceProductBaseCode=AE
  Quaternion Rotation : aerolibutil/Quaternion Rotation
  Vector Concatenate3 : Concatenate  NumInputs=3
  Out1 : Outport
  wires:
  Quaternion Conjugate1/1 -> Quaternion Rotation/1
  Data Type Conversion4/1 -> Demux1/1
  Mux1/1 -> Out1/1
  Mux/1 -> Quaternion Conjugate1/1, Mux1/4
  Add3/1 -> Mux1/3
  Add2/1 -> Mux1/2
  Add1/1 -> Mux1/1
  Demux/7 -> Mux/4
  Demux/6 -> Mux/3
  Demux/5 -> Mux/2
  Demux/4 -> Mux/1
  In1/1 -> Demux/1
  In4/1 -> Vector Concatenate3/3
  Demux/1 -> Add1/1
  In3/1 -> Vector Concatenate3/2
  Demux/3 -> Add3/1
  Quaternion Rotation/1 -> Data Type Conversion4/1
  Demux1/3 -> Add3/2
  Vector Concatenate3/1 -> Quaternion Rotation/2
  Demux1/2 -> Add2/2
  Demux1/1 -> Add1/2
  In2/1 -> Vector Concatenate3/1
  Demux/2 -> Add2/1

== system W02_Base_Map_PB_cs/BMW_X5_SUV_1/move_base_simple//goal ==
  In1 : Inport
  Enable : EnablePort
  Add4 : Sum
  Assignment4 : Assignment  OutputInitialize=Specify size for each dimension in table  DiagnosticForDimensions=Warning  IndexOptions=Starting index (dialog)  Indices=1  OutputSizes=1000
  Blank Message5 : robotlib/Blank Message  messageClass=Message  entityType=geometry_msgs/PoseStamped  messageType=geometry_msgs/PoseStamped  SampleTime=inf
      settings: SourceProductBaseCode=RO
  Bus Assignment4 : BusAssignment  AssignedSignals=Header.Seq,Header.FrameId,Header.FrameId_SL_Info.CurrentLength,Pose.Position.X,Pose.Position.Y,Pose.Position.Z,Pose.Orientation.W,Pose.Orientation.X,Pose.Orientation.Y,Pose.Orientation.Z
  Bus Selector3 : BusSelector  OutputSignals=Header.FrameId
  Constant8 : Constant  OutDataTypeStr=uint32
  Constant9 : Constant  Value=uint8(['world'])
  Demux : Demux  Outputs=7
  Memory1 : Memory  InheritSampleTime=on
  Publish1 : robotlib/Publish  topicSource=Select from ROS network  topic=/move_base_simple/goal  messageType=geometry_msgs/PoseStamped  messageQueueLength=1
      settings: SourceProductBaseCode=RO
  Width4 : Width  DataType=uint32
  wires:
  Demux/7 -> Bus Assignment4/11
  Demux/6 -> Bus Assignment4/10
  Demux/5 -> Bus Assignment4/9
  Demux/4 -> Bus Assignment4/8
  Demux/3 -> Bus Assignment4/7
  Demux/2 -> Bus Assignment4/6
  Demux/1 -> Bus Assignment4/5
  In1/1 -> Demux/1
  Width4/1 -> Bus Assignment4/4
  Memory1/1 -> Add4/1
  Constant9/1 -> Width4/1, Assignment4/2
  Constant8/1 -> Add4/2
  Bus Assignment4/1 -> Publish1/1
  Bus Selector3/1 -> Assignment4/1  "<FrameId>"
  Assignment4/1 -> Bus Assignment4/3
  Add4/1 -> Memory1/1, Bus Assignment4/2
  Blank Message5/1 -> Bus Assignment4/1, Bus Selector3/1

== system W02_Base_Map_PB_cs/BMW_X5_SUV_1/tl_camera_CM_Demux ==
  In1 : Inport
  Selector : Selector  NumberOfDimensions=2  InputPortWidth=3  IndexOptions=Index vector (dialog),Index vector (dialog)  Indices=-1,1:hres  OutputSizes=1,1
  Selector1 : Selector  NumberOfDimensions=2  InputPortWidth=3  IndexOptions=Index vector (dialog),Index vector (dialog)  Indices=-1,hres+1:hres*2  OutputSizes=1,1
  Selector2 : Selector  NumberOfDimensions=2  InputPortWidth=3  IndexOptions=Index vector (dialog),Index vector (dialog)  Indices=-1,hres*2+1:hres*3  OutputSizes=1,1
  R : Outport
  G : Outport  Port=2
  B : Outport  Port=3
  wires:
  In1/1 -> Selector1/1, Selector/1, Selector2/1
  Selector/1 -> R/1
  Selector1/1 -> G/1
  Selector2/1 -> B/1

== system W02_Base_Map_PB_cs/BMW_X5_SUV_1/tonemap ==
  In1 : Inport
  Constant : Constant  Value=255
  Data Type Conversion : DataTypeConversion  OutDataTypeStr=uint8
  Product : Product
  Square Root : Sqrt  SaturateOnIntegerOverflow=on
  Out1 : Outport
  wires:
  In1/1 -> Square Root/1
  Square Root/1 -> Product/1
  Product/1 -> Data Type Conversion/1
  Constant/1 -> Product/2
  Data Type Conversion/1 -> Out1/1

== system W02_Base_Map_PB_cs/Citroen_C3_Hatchback_1/AIR_2_Demux ==
  AIR : Inport
  Activate_Switch : Subsystem
      mask Display: text(5,10,'')
  Bus Selector : BusSelector  OutputSignals=DATA.Range,DATA.Azimuth,DATA.Elevation,DATA.ID,DATA.Velocity,DATA.Heading
  Data Type Conversion : DataTypeConversion  OutDataTypeStr=double
  For Iterator : ForIterator  ResetStates=reset  IterationLimit=detectableObjects
  Selector : Selector  InputPortWidth=detectableObjects  IndexOptions=Index vector (port)  Indices=[1 3]  OutputSizes=1
  Signal2ArrayOfSignals1 : Subsystem  mask{VECTORLENGTH=detectableObjects}
      mask prompts: VECTORLENGTH "Length of vector"
  Signal2ArrayOfSignals2 : Subsystem  mask{VECTORLENGTH=detectableObjects}
      mask prompts: VECTORLENGTH "Length of vector"
  Signal2ArrayOfSignals3 : Subsystem  mask{VECTORLENGTH=detectableObjects}
      mask prompts: VECTORLENGTH "Length of vector"
  Signal2ArrayOfSignals4 : Subsystem  mask{VECTORLENGTH=detectableObjects}
      mask prompts: VECTORLENGTH "Length of vector"
  Signal2ArrayOfSignals5 : Subsystem  mask{VECTORLENGTH=detectableObjects}
      mask prompts: VECTORLENGTH "Length of vector"
  Signal2ArrayOfSignals6 : Subsystem  mask{VECTORLENGTH=detectableObjects}
      mask prompts: VECTORLENGTH "Length of vector"
  Range [m] : Outport
  Azimuth [deg] : Outport  Port=2
  Elevation [deg] : Outport  Port=3
  ID [-] : Outport  Port=4
  Velocity [m/s] : Outport  Port=5
  Heading [deg] : Outport  Port=6
  wires:
  Data Type Conversion/1 -> ID [-]/1
  Bus Selector/6 -> Signal2ArrayOfSignals6/2(Element)  "<Heading>"
  Signal2ArrayOfSignals6/1(ArrayofElements) -> Activate_Switch/2(Heading)
  Bus Selector/5 -> Signal2ArrayOfSignals5/2(Element)  "<Velocity>"
  Signal2ArrayOfSignals5/1(ArrayofElements) -> Velocity [m/s]/1
  Bus Selector/4 -> Signal2ArrayOfSignals4/2(Element)  "<ID>"
  Signal2ArrayOfSignals4/1(ArrayofElements) -> Data Type Conversion/1, Activate_Switch/1(BeamID)
  Bus Selector/3 -> Signal2ArrayOfSignals3/2(Element)  "<Elevation>"
  Signal2ArrayOfSignals3/1(ArrayofElements) -> Elevation [deg]/1
  Bus Selector/2 -> Signal2ArrayOfSignals1/2(Element)  "<Azimuth>"
  Signal2ArrayOfSignals1/1(ArrayofElements) -> Azimuth [deg]/1
  Signal2ArrayOfSignals2/1(ArrayofElements) -> Range [m]/1
  Bus Selector/1 -> Signal2ArrayOfSignals2/2(Element)  "<Range>"
  Selector/1 -> Bus Selector/1
  For Iterator/1 -> Signal2ArrayOfSignals6/1(LoopIndex), Signal2ArrayOfSignals5/1(LoopIndex), Signal2ArrayOfSignals4/1(LoopIndex), Signal2ArrayOfSignals3/1(LoopIndex), Signal2ArrayOfSignals1/1(LoopIndex), Signal2ArrayOfSignals2/1(LoopIndex), Selector/2
  AIR/1 -> Selector/1
  Activate_Switch/1(On/Off) -> Heading [deg]/1
